simulink model "motor_model"  (R2015a)
settings: Solver=ode45  StartTime=0.0  StopTime=10.0  RelTol=1e-3
undefined symbols (not defined in the file or in its folder): magnitude
settings Model: Creator=Paul  LastModifiedBy=Paul

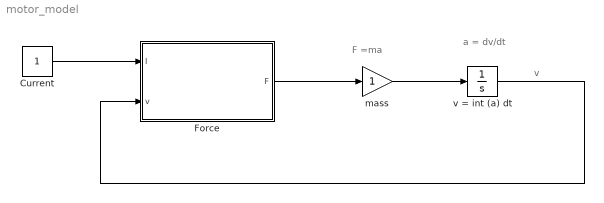
== system motor_model ==
  note: v
  note: F =ma
  note: a = dv/dt
  Current : Constant
  "Force " : Subsystem
  mass : Gain
  v = int (a) dt : Integrator
  wires:
  mass/1 -> v = int (a) dt/1
  v = int (a) dt/1 -> "Force "/2(v)
  "Force "/1("F ") -> mass/1
  Current/1 -> "Force "/1("I ")

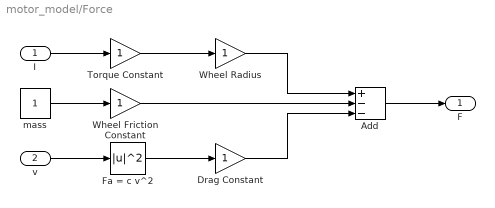
== system motor_model/Force  ==
  "I " : Inport
  v : Inport  Port=2
  Add : Sum  Inputs=+--
  Drag Constant : Gain
  "Fa = c v^2 " : Math  Operator=magnitude^2  SaturateOnIntegerOverflow=on
  Torque Constant : Gain
  Wheel Friction Constant : Gain
  Wheel Radius : Gain
  "mass " : Constant
  "F " : Outport
  wires:
  Add/1 -> "F "/1
  v/1 -> "Fa = c v^2 "/1
  "Fa = c v^2 "/1 -> Drag Constant/1
  Wheel Friction Constant/1 -> Add/2
  "mass "/1 -> Wheel Friction Constant/1
  Torque Constant/1 -> Wheel Radius/1
  Wheel Radius/1 -> Add/1
  "I "/1 -> Torque Constant/1
  Drag Constant/1 -> Add/3
